simulink model "Project_Papi_Rubber_Game_LeastNorm_Sim"  (R2019a)
settings: Solver=FixedStepAuto  StartTime=0.0  StopTime=50.0  FixedStep=0.01  RelTol=1e-3
values from neighbouring files (symbols this model uses):
  A = [0 0 0 0 0 0 ... (first row only)    [Final_Code.m]
  B = [1 0 ... (first row only)    [Final_Code.m]
  C = [1 0 0 0 0 0 ... (first row only)    [Final_Code.m]
  ene = [ene4(1,1)+(dia3/2) ene4(1,2)+(dia3/2)]    [Final_Code.m]
  init_cond = [out.x_plant.Data(j,1); out.x_plant.Data(j,2); out.x_plant.Data(j,3); out.x_plant.Data(j,4); out.x_plant.Data(j,5); out.x_plant.Data(j,6)]    [Final_Code.m]
  m = 1    [Final_Code.m]
  R = 300    [Final_Code.m]
  slop = [2 -1 3 -2]    [Final_Code.m]
undefined symbols (not defined in the file or in its folder): phi
libraries: simulink x2, dspinverses x1
settings Model: Creator=asjos  LastModifiedBy=asjos

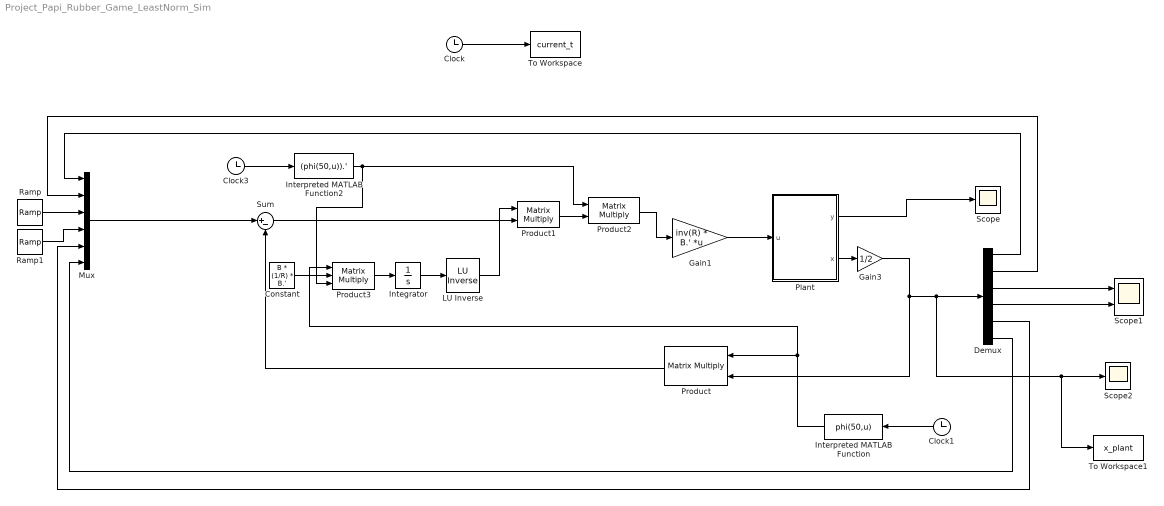
== system Project_Papi_Rubber_Game_LeastNorm_Sim ==
  " LU Inverse" : dspinverses/ LU Inverse
      settings: SourceProductName=DSP System Toolbox
  Clock : Clock
  Clock1 : Clock
  Clock3 : Clock
  Constant : Constant  Value=B * (1/R) * B.'
  Demux : Demux  Outputs=6
  Gain1 : Gain  Gain=inv(R) * B.'  Multiplication=Matrix(K*u)
  Gain3 : Gain  Gain=1/2
  Integrator : Integrator  InitialCondition=eye(6)
  Interpreted MATLAB Function : MATLABFcn  MATLABFcn=phi(50,u)  Output1D=off
  Interpreted MATLAB Function2 : MATLABFcn  MATLABFcn=(phi(50,u)).'  Output1D=off
  Mux : Mux  Inputs=6
  Plant : Subsystem
  Product : Product  Multiplication=Matrix(*)
  Product1 : Product  Multiplication=Matrix(*)
  Product2 : Product  Multiplication=Matrix(*)
  Product3 : Product  Inputs=3  Multiplication=Matrix(*)
  Ramp : simulink/Sources/Ramp  slope=slop(1,m)  start=0  InitialOutput=ene(1,1)
  Ramp1 : simulink/Sources/Ramp  slope=slop(1,m)  start=0  InitialOutput=ene(1,2)
  Scope : Scope
  Scope1 : Scope  NumInputPorts=2
  Scope2 : Scope
  Sum : Sum  Inputs=|+-
  To Workspace : ToWorkspace  VariableName=current_t  SampleTime=-1
  To Workspace1 : ToWorkspace  VariableName=x_plant  SaveFormat=Timeseries  SampleTime=-1
  wires:
  Clock/1 -> To Workspace/1
  Clock1/1 -> Interpreted MATLAB Function/1
  Product/1 -> Sum/2
  Interpreted MATLAB Function/1 -> Product3/1, Product/1
  Plant/2(x) -> Gain3/1
  Clock3/1 -> Interpreted MATLAB Function2/1
  Product2/1 -> Gain1/1
  Gain1/1 -> Plant/1(u)
  Demux/4 -> Scope1/2
  Demux/3 -> Scope1/1
  Sum/1 -> Product1/2
  Interpreted MATLAB Function2/1 -> Product3/3, Product2/1
  Product1/1 -> Product2/2
  Constant/1 -> Product3/2
  Product3/1 -> Integrator/1
  Integrator/1 -> " LU Inverse"/1
  " LU Inverse"/1 -> Product1/1
  Demux/5 -> Mux/5
  Demux/6 -> Mux/6
  Demux/1 -> Mux/1
  Demux/2 -> Mux/2
  Ramp/1 -> Mux/3
  Ramp1/1 -> Mux/4
  Mux/1 -> Sum/1
  Plant/1(y) -> Scope/1
  Gain3/1 -> To Workspace1/1, Scope2/1, Demux/1, Product/2

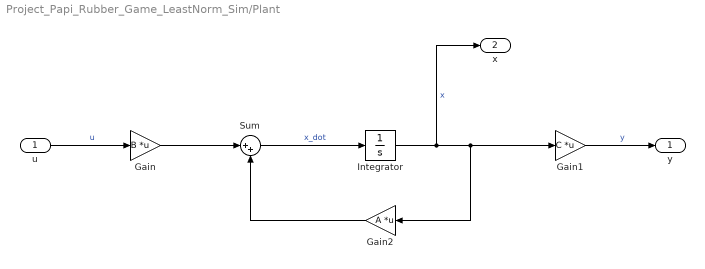
== system Project_Papi_Rubber_Game_LeastNorm_Sim/Plant ==
  u : Inport
  Gain : Gain  Gain=B  Multiplication=Matrix(K*u)
  Gain1 : Gain  Gain=C  Multiplication=Matrix(K*u)
  Gain2 : Gain  Gain=A  Multiplication=Matrix(K*u)
  Integrator : Integrator  InitialCondition=init_cond
  Sum : Sum  Inputs=|++
  y : Outport
  x : Outport  Port=2
  wires:
  Integrator/1 -> x/1, Gain1/1, Gain2/1  "x"
  Gain2/1 -> Sum/2
  Gain/1 -> Sum/1
  Sum/1 -> Integrator/1  "x_dot"
  u/1 -> Gain/1  "u"
  Gain1/1 -> y/1  "y"
